simulink model "CMNot_Model"  (R2024b)
settings: Solver=VariableStepAuto  StartTime=0.0  StopTime=10.0  RelTol=1e-3
libraries: NSA_DEVS_SINKS x2, NSA_DEVS_LOGISTICS x1, NSA_DEVS_SOURCES x1, NSA_DEVS_DIGITAL_LOGIC x1
settings Model: Creator=david  LastModifiedBy=peter
settings RTWCC: GPUComputeCapability=3.5

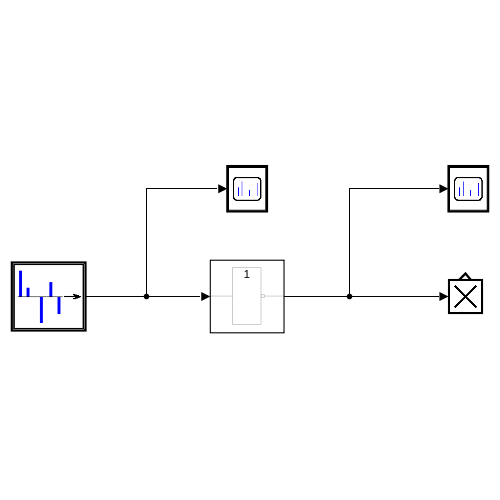
[thumbnail: Simulink's stored preview of the top-level diagram]
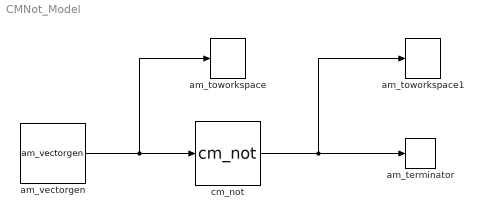
== system CMNot_Model ==
  am_terminator : NSA_DEVS_LOGISTICS/am_terminator  tau=[0,1]  debug=0
      settings: SourceProductName=Logistics
  am_toworkspace : NSA_DEVS_SINKS/am_toworkspace  varname="\"gen1Out\""  t0=0  format="\"vector\""  tau=[0,5]  debug=0
      settings: SourceProductName=Sinks
  am_toworkspace1 : NSA_DEVS_SINKS/am_toworkspace  varname="\"notOut\""  t0=0  format="\"vector\""  tau=[0,5]  debug=0
      settings: SourceProductName=Sinks
  am_vectorgen : NSA_DEVS_SOURCES/am_vectorgen  tvec="[0,   1,  2,  3]"  yvec="[\"0\",\"1\",\"0\",\"1\"]"  tau=[0,1]  debug=0
      settings: SourceProductName=Sources
  cm_not : NSA_DEVS_DIGITAL_LOGIC/cm_not  tau=[0,1]  debug=0
      settings: SourceProductName=Logic
  wires:
  am_vectorgen/1 -> am_toworkspace/1, cm_not/1
  cm_not/1 -> am_toworkspace1/1, am_terminator/1
